simulink model "simulacion_profe_trim"  (R2024a)
settings: Solver=VariableStepAuto  StartTime=0.0  StopTime=10.0  RelTol=1e-3
settings Model: Creator=damia  LastModifiedBy=damia

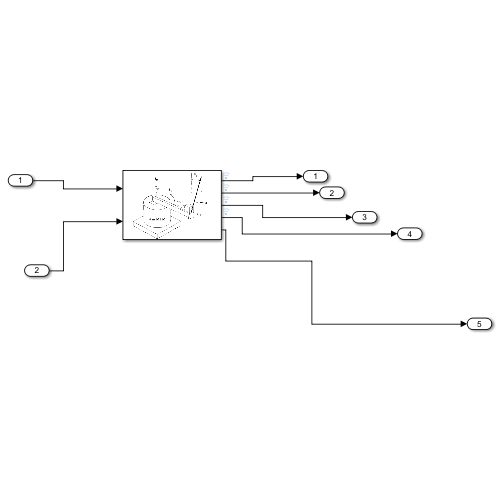
[thumbnail: Simulink's stored preview of the top-level diagram]
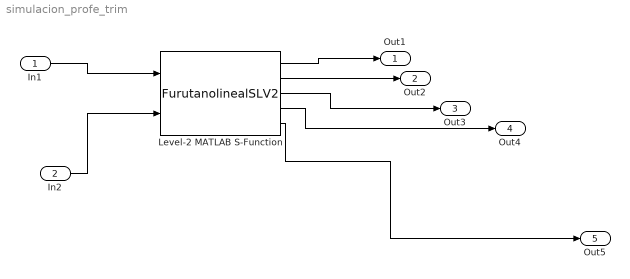
== system simulacion_profe_trim ==
  In1 : Inport
  In2 : Inport  Port=2
  Level-2 MATLAB S-Function : M-S-Function  FunctionName=FurutanolinealSLV2  mask{Xi=0, g=0, J=0, M_2=0, l_bi=0, C_x=0, C_z=0, I_x=0, I_z=0}
      mask prompts: Xi "Parametros iniciales (Xi)"
      mask Display: image('mascara2.png');
  Out1 : Outport
  Out2 : Outport  Port=2
  Out3 : Outport  Port=3
  Out4 : Outport  Port=4
  Out5 : Outport  Port=5
  wires:
  In1/1 -> Level-2 MATLAB S-Function/1
  In2/1 -> Level-2 MATLAB S-Function/2
  Level-2 MATLAB S-Function/1 -> Out1/1
  Level-2 MATLAB S-Function/2 -> Out2/1
  Level-2 MATLAB S-Function/3 -> Out3/1
  Level-2 MATLAB S-Function/4 -> Out4/1
  Level-2 MATLAB S-Function/5 -> Out5/1
